simulink model "PROGRAM_COUNTER_05_SS"  (R2022a)
settings: Solver=VariableStepAuto  StartTime=0.0  StopTime=10.0  RelTol=1e-3
undefined symbols (not defined in the file or in its folder): xc7z010iclg225
libraries: hdlBasic x1928, hlsBasic x1, vmcUtilities x1
(part 3 of 12)

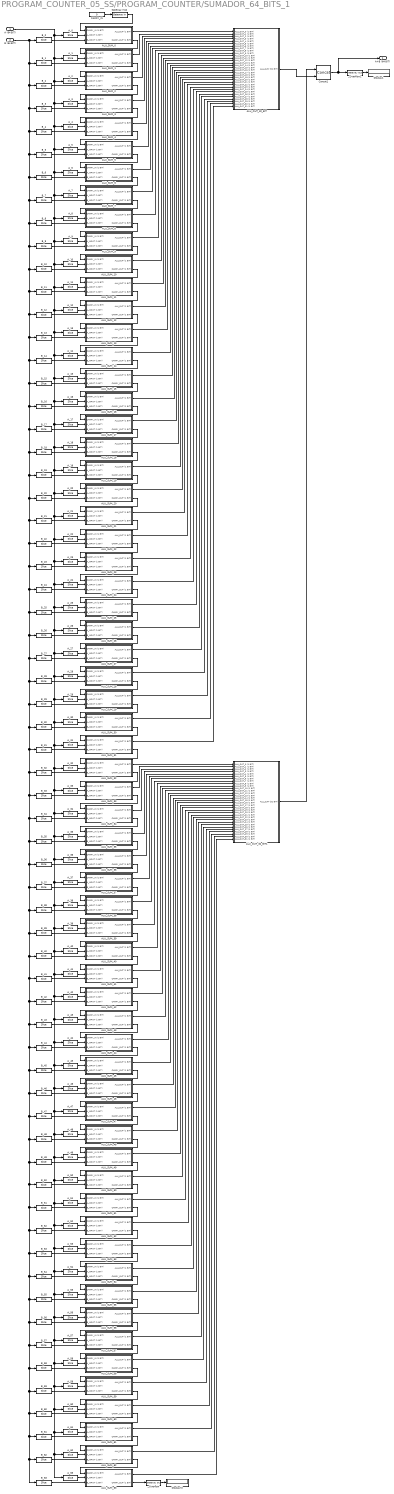
== system PROGRAM_COUNTER_05_SS/PROGRAM_COUNTER/SUMADOR_64_BITS_1 ==
  A (64 BIT) : Inport
  B (64 BIT) : Inport  Port=2
  ALU_OUT_32_BIT : Subsystem
  ALU_OUT_32_BIT1 : Subsystem
  ALU_SUM_0 : Subsystem
  ALU_SUM_1 : Subsystem
  ALU_SUM_10 : Subsystem
  ALU_SUM_11 : Subsystem
  ALU_SUM_12 : Subsystem
  ALU_SUM_13 : Subsystem
  ALU_SUM_14 : Subsystem
  ALU_SUM_15 : Subsystem
  ALU_SUM_16 : Subsystem
  ALU_SUM_17 : Subsystem
  ALU_SUM_18 : Subsystem
  ALU_SUM_19 : Subsystem
  ALU_SUM_2 : Subsystem
  ALU_SUM_20 : Subsystem
  ALU_SUM_21 : Subsystem
  ALU_SUM_22 : Subsystem
  ALU_SUM_23 : Subsystem
  ALU_SUM_24 : Subsystem
  ALU_SUM_25 : Subsystem
  ALU_SUM_26 : Subsystem
  ALU_SUM_27 : Subsystem
  ALU_SUM_28 : Subsystem
  ALU_SUM_29 : Subsystem
  ALU_SUM_3 : Subsystem
  ALU_SUM_30 : Subsystem
  ALU_SUM_31 : Subsystem
  ALU_SUM_32 : Subsystem
  ALU_SUM_33 : Subsystem
  ALU_SUM_34 : Subsystem
  ALU_SUM_35 : Subsystem
  ALU_SUM_36 : Subsystem
  ALU_SUM_37 : Subsystem
  ALU_SUM_38 : Subsystem
  ALU_SUM_39 : Subsystem
  ALU_SUM_4 : Subsystem
  ALU_SUM_40 : Subsystem
  ALU_SUM_41 : Subsystem
  ALU_SUM_42 : Subsystem
  ALU_SUM_43 : Subsystem
  ALU_SUM_44 : Subsystem
  ALU_SUM_45 : Subsystem
  ALU_SUM_46 : Subsystem
  ALU_SUM_47 : Subsystem
  ALU_SUM_48 : Subsystem
  ALU_SUM_49 : Subsystem
  ALU_SUM_5 : Subsystem
  ALU_SUM_50 : Subsystem
  ALU_SUM_51 : Subsystem
  ALU_SUM_52 : Subsystem
  ALU_SUM_53 : Subsystem
  ALU_SUM_54 : Subsystem
  ALU_SUM_55 : Subsystem
  ALU_SUM_56 : Subsystem
  ALU_SUM_57 : Subsystem
  ALU_SUM_58 : Subsystem
  ALU_SUM_59 : Subsystem
  ALU_SUM_6 : Subsystem
  ALU_SUM_60 : Subsystem
  ALU_SUM_61 : Subsystem
  ALU_SUM_62 : Subsystem
  ALU_SUM_63 : Subsystem
  ALU_SUM_7 : Subsystem
  ALU_SUM_8 : Subsystem
  ALU_SUM_9 : Subsystem
  A_0 : hdlBasic/Slice  nbits=1  boolean_output=off  mode=Lower Bit Location + Width  bit1=-3  base1=MSB of Input  bit0=0  base0=LSB of Input  XmcBlockStatus=1  maskContainerNames=group1  block_type=slice  block_config=sysgen:Slice_config
  A_1 : hdlBasic/Slice  nbits=1  boolean_output=off  mode=Lower Bit Location + Width  bit1=-2  base1=MSB of Input  bit0=1  base0=LSB of Input  XmcBlockStatus=1  maskContainerNames=group1  block_type=slice  block_config=sysgen:Slice_config
  A_10 : hdlBasic/Slice  nbits=1  boolean_output=off  mode=Lower Bit Location + Width  bit1=-1  base1=MSB of Input  bit0=10  base0=LSB of Input  XmcBlockStatus=1  maskContainerNames=group1  block_type=slice  block_config=sysgen:Slice_config
  A_11 : hdlBasic/Slice  nbits=1  boolean_output=off  mode=Lower Bit Location + Width  bit1=-3  base1=MSB of Input  bit0=11  base0=LSB of Input  XmcBlockStatus=1  maskContainerNames=group1  block_type=slice  block_config=sysgen:Slice_config
  A_12 : hdlBasic/Slice  nbits=1  boolean_output=off  mode=Lower Bit Location + Width  bit1=-2  base1=MSB of Input  bit0=12  base0=LSB of Input  XmcBlockStatus=1  maskContainerNames=group1  block_type=slice  block_config=sysgen:Slice_config
  A_13 : hdlBasic/Slice  nbits=1  boolean_output=off  mode=Lower Bit Location + Width  bit1=-1  base1=MSB of Input  bit0=13  base0=LSB of Input  XmcBlockStatus=1  maskContainerNames=group1  block_type=slice  block_config=sysgen:Slice_config
  A_14 : hdlBasic/Slice  nbits=1  boolean_output=off  mode=Lower Bit Location + Width  bit1=-1  base1=MSB of Input  bit0=14  base0=LSB of Input  XmcBlockStatus=1  maskContainerNames=group1  block_type=slice  block_config=sysgen:Slice_config
  A_15 : hdlBasic/Slice  nbits=1  boolean_output=off  mode=Lower Bit Location + Width  bit1=-3  base1=MSB of Input  bit0=15  base0=LSB of Input  XmcBlockStatus=1  maskContainerNames=group1  block_type=slice  block_config=sysgen:Slice_config
  A_16 : hdlBasic/Slice  nbits=1  boolean_output=off  mode=Lower Bit Location + Width  bit1=-2  base1=MSB of Input  bit0=16  base0=LSB of Input  XmcBlockStatus=1  maskContainerNames=group1  block_type=slice  block_config=sysgen:Slice_config
  A_17 : hdlBasic/Slice  nbits=1  boolean_output=off  mode=Lower Bit Location + Width  bit1=-1  base1=MSB of Input  bit0=17  base0=LSB of Input  XmcBlockStatus=1  maskContainerNames=group1  block_type=slice  block_config=sysgen:Slice_config
  A_18 : hdlBasic/Slice  nbits=1  boolean_output=off  mode=Lower Bit Location + Width  bit1=-1  base1=MSB of Input  bit0=18  base0=LSB of Input  XmcBlockStatus=1  maskContainerNames=group1  block_type=slice  block_config=sysgen:Slice_config
  A_19 : hdlBasic/Slice  nbits=1  boolean_output=off  mode=Lower Bit Location + Width  bit1=-3  base1=MSB of Input  bit0=19  base0=LSB of Input  XmcBlockStatus=1  maskContainerNames=group1  block_type=slice  block_config=sysgen:Slice_config
  A_2 : hdlBasic/Slice  nbits=1  boolean_output=off  mode=Lower Bit Location + Width  bit1=-1  base1=MSB of Input  bit0=2  base0=LSB of Input  XmcBlockStatus=1  maskContainerNames=group1  block_type=slice  block_config=sysgen:Slice_config
  A_20 : hdlBasic/Slice  nbits=1  boolean_output=off  mode=Lower Bit Location + Width  bit1=-2  base1=MSB of Input  bit0=20  base0=LSB of Input  XmcBlockStatus=1  maskContainerNames=group1  block_type=slice  block_config=sysgen:Slice_config
  A_21 : hdlBasic/Slice  nbits=1  boolean_output=off  mode=Lower Bit Location + Width  bit1=-1  base1=MSB of Input  bit0=21  base0=LSB of Input  XmcBlockStatus=1  maskContainerNames=group1  block_type=slice  block_config=sysgen:Slice_config
  A_22 : hdlBasic/Slice  nbits=1  boolean_output=off  mode=Lower Bit Location + Width  bit1=-1  base1=MSB of Input  bit0=22  base0=LSB of Input  XmcBlockStatus=1  maskContainerNames=group1  block_type=slice  block_config=sysgen:Slice_config
  A_23 : hdlBasic/Slice  nbits=1  boolean_output=off  mode=Lower Bit Location + Width  bit1=-3  base1=MSB of Input  bit0=23  base0=LSB of Input  XmcBlockStatus=1  maskContainerNames=group1  block_type=slice  block_config=sysgen:Slice_config
  A_24 : hdlBasic/Slice  nbits=1  boolean_output=off  mode=Lower Bit Location + Width  bit1=-2  base1=MSB of Input  bit0=24  base0=LSB of Input  XmcBlockStatus=1  maskContainerNames=group1  block_type=slice  block_config=sysgen:Slice_config
  A_25 : hdlBasic/Slice  nbits=1  boolean_output=off  mode=Lower Bit Location + Width  bit1=-1  base1=MSB of Input  bit0=25  base0=LSB of Input  XmcBlockStatus=1  maskContainerNames=group1  block_type=slice  block_config=sysgen:Slice_config
  A_26 : hdlBasic/Slice  nbits=1  boolean_output=off  mode=Lower Bit Location + Width  bit1=-1  base1=MSB of Input  bit0=26  base0=LSB of Input  XmcBlockStatus=1  maskContainerNames=group1  block_type=slice  block_config=sysgen:Slice_config
  A_27 : hdlBasic/Slice  nbits=1  boolean_output=off  mode=Lower Bit Location + Width  bit1=-3  base1=MSB of Input  bit0=27  base0=LSB of Input  XmcBlockStatus=1  maskContainerNames=group1  block_type=slice  block_config=sysgen:Slice_config
  A_28 : hdlBasic/Slice  nbits=1  boolean_output=off  mode=Lower Bit Location + Width  bit1=-2  base1=MSB of Input  bit0=28  base0=LSB of Input  XmcBlockStatus=1  maskContainerNames=group1  block_type=slice  block_config=sysgen:Slice_config
  A_29 : hdlBasic/Slice  nbits=1  boolean_output=off  mode=Lower Bit Location + Width  bit1=-1  base1=MSB of Input  bit0=29  base0=LSB of Input  XmcBlockStatus=1  maskContainerNames=group1  block_type=slice  block_config=sysgen:Slice_config
  A_3 : hdlBasic/Slice  nbits=1  boolean_output=off  mode=Lower Bit Location + Width  bit1=-3  base1=MSB of Input  bit0=3  base0=LSB of Input  XmcBlockStatus=1  maskContainerNames=group1  block_type=slice  block_config=sysgen:Slice_config
  A_30 : hdlBasic/Slice  nbits=1  boolean_output=off  mode=Lower Bit Location + Width  bit1=-1  base1=MSB of Input  bit0=30  base0=LSB of Input  XmcBlockStatus=1  maskContainerNames=group1  block_type=slice  block_config=sysgen:Slice_config
  A_31 : hdlBasic/Slice  nbits=1  boolean_output=off  mode=Lower Bit Location + Width  bit1=-3  base1=MSB of Input  bit0=31  base0=LSB of Input  XmcBlockStatus=1  maskContainerNames=group1  block_type=slice  block_config=sysgen:Slice_config
  A_32 : hdlBasic/Slice  nbits=1  boolean_output=off  mode=Lower Bit Location + Width  bit1=-1  base1=MSB of Input  bit0=32  base0=LSB of Input  XmcBlockStatus=1  maskContainerNames=group1  block_type=slice  block_config=sysgen:Slice_config
  A_33 : hdlBasic/Slice  nbits=1  boolean_output=off  mode=Lower Bit Location + Width  bit1=-3  base1=MSB of Input  bit0=33  base0=LSB of Input  XmcBlockStatus=1  maskContainerNames=group1  block_type=slice  block_config=sysgen:Slice_config
  A_34 : hdlBasic/Slice  nbits=1  boolean_output=off  mode=Lower Bit Location + Width  bit1=-1  base1=MSB of Input  bit0=34  base0=LSB of Input  XmcBlockStatus=1  maskContainerNames=group1  block_type=slice  block_config=sysgen:Slice_config
  A_35 : hdlBasic/Slice  nbits=1  boolean_output=off  mode=Lower Bit Location + Width  bit1=-3  base1=MSB of Input  bit0=35  base0=LSB of Input  XmcBlockStatus=1  maskContainerNames=group1  block_type=slice  block_config=sysgen:Slice_config
  A_36 : hdlBasic/Slice  nbits=1  boolean_output=off  mode=Lower Bit Location + Width  bit1=-1  base1=MSB of Input  bit0=36  base0=LSB of Input  XmcBlockStatus=1  maskContainerNames=group1  block_type=slice  block_config=sysgen:Slice_config
  A_37 : hdlBasic/Slice  nbits=1  boolean_output=off  mode=Lower Bit Location + Width  bit1=-3  base1=MSB of Input  bit0=37  base0=LSB of Input  XmcBlockStatus=1  maskContainerNames=group1  block_type=slice  block_config=sysgen:Slice_config
  A_38 : hdlBasic/Slice  nbits=1  boolean_output=off  mode=Lower Bit Location + Width  bit1=-1  base1=MSB of Input  bit0=38  base0=LSB of Input  XmcBlockStatus=1  maskContainerNames=group1  block_type=slice  block_config=sysgen:Slice_config
  A_39 : hdlBasic/Slice  nbits=1  boolean_output=off  mode=Lower Bit Location + Width  bit1=-3  base1=MSB of Input  bit0=39  base0=LSB of Input  XmcBlockStatus=1  maskContainerNames=group1  block_type=slice  block_config=sysgen:Slice_config
  A_4 : hdlBasic/Slice  nbits=1  boolean_output=off  mode=Lower Bit Location + Width  bit1=-2  base1=MSB of Input  bit0=4  base0=LSB of Input  XmcBlockStatus=1  maskContainerNames=group1  block_type=slice  block_config=sysgen:Slice_config
  A_40 : hdlBasic/Slice  nbits=1  boolean_output=off  mode=Lower Bit Location + Width  bit1=-1  base1=MSB of Input  bit0=40  base0=LSB of Input  XmcBlockStatus=1  maskContainerNames=group1  block_type=slice  block_config=sysgen:Slice_config
  A_41 : hdlBasic/Slice  nbits=1  boolean_output=off  mode=Lower Bit Location + Width  bit1=-3  base1=MSB of Input  bit0=41  base0=LSB of Input  XmcBlockStatus=1  maskContainerNames=group1  block_type=slice  block_config=sysgen:Slice_config
  A_42 : hdlBasic/Slice  nbits=1  boolean_output=off  mode=Lower Bit Location + Width  bit1=-1  base1=MSB of Input  bit0=42  base0=LSB of Input  XmcBlockStatus=1  maskContainerNames=group1  block_type=slice  block_config=sysgen:Slice_config
  A_43 : hdlBasic/Slice  nbits=1  boolean_output=off  mode=Lower Bit Location + Width  bit1=-3  base1=MSB of Input  bit0=43  base0=LSB of Input  XmcBlockStatus=1  maskContainerNames=group1  block_type=slice  block_config=sysgen:Slice_config
  A_44 : hdlBasic/Slice  nbits=1  boolean_output=off  mode=Lower Bit Location + Width  bit1=-1  base1=MSB of Input  bit0=44  base0=LSB of Input  XmcBlockStatus=1  maskContainerNames=group1  block_type=slice  block_config=sysgen:Slice_config
  A_45 : hdlBasic/Slice  nbits=1  boolean_output=off  mode=Lower Bit Location + Width  bit1=-3  base1=MSB of Input  bit0=45  base0=LSB of Input  XmcBlockStatus=1  maskContainerNames=group1  block_type=slice  block_config=sysgen:Slice_config
  A_46 : hdlBasic/Slice  nbits=1  boolean_output=off  mode=Lower Bit Location + Width  bit1=-1  base1=MSB of Input  bit0=46  base0=LSB of Input  XmcBlockStatus=1  maskContainerNames=group1  block_type=slice  block_config=sysgen:Slice_config
  A_47 : hdlBasic/Slice  nbits=1  boolean_output=off  mode=Lower Bit Location + Width  bit1=-3  base1=MSB of Input  bit0=47  base0=LSB of Input  XmcBlockStatus=1  maskContainerNames=group1  block_type=slice  block_config=sysgen:Slice_config
  A_48 : hdlBasic/Slice  nbits=1  boolean_output=off  mode=Lower Bit Location + Width  bit1=-1  base1=MSB of Input  bit0=48  base0=LSB of Input  XmcBlockStatus=1  maskContainerNames=group1  block_type=slice  block_config=sysgen:Slice_config
  A_49 : hdlBasic/Slice  nbits=1  boolean_output=off  mode=Lower Bit Location + Width  bit1=-3  base1=MSB of Input  bit0=49  base0=LSB of Input  XmcBlockStatus=1  maskContainerNames=group1  block_type=slice  block_config=sysgen:Slice_config
  A_5 : hdlBasic/Slice  nbits=1  boolean_output=off  mode=Lower Bit Location + Width  bit1=-1  base1=MSB of Input  bit0=5  base0=LSB of Input  XmcBlockStatus=1  maskContainerNames=group1  block_type=slice  block_config=sysgen:Slice_config
  A_50 : hdlBasic/Slice  nbits=1  boolean_output=off  mode=Lower Bit Location + Width  bit1=-1  base1=MSB of Input  bit0=50  base0=LSB of Input  XmcBlockStatus=1  maskContainerNames=group1  block_type=slice  block_config=sysgen:Slice_config
  A_51 : hdlBasic/Slice  nbits=1  boolean_output=off  mode=Lower Bit Location + Width  bit1=-3  base1=MSB of Input  bit0=51  base0=LSB of Input  XmcBlockStatus=1  maskContainerNames=group1  block_type=slice  block_config=sysgen:Slice_config
  A_52 : hdlBasic/Slice  nbits=1  boolean_output=off  mode=Lower Bit Location + Width  bit1=-1  base1=MSB of Input  bit0=52  base0=LSB of Input  XmcBlockStatus=1  maskContainerNames=group1  block_type=slice  block_config=sysgen:Slice_config
  A_53 : hdlBasic/Slice  nbits=1  boolean_output=off  mode=Lower Bit Location + Width  bit1=-3  base1=MSB of Input  bit0=53  base0=LSB of Input  XmcBlockStatus=1  maskContainerNames=group1  block_type=slice  block_config=sysgen:Slice_config
  A_54 : hdlBasic/Slice  nbits=1  boolean_output=off  mode=Lower Bit Location + Width  bit1=-1  base1=MSB of Input  bit0=54  base0=LSB of Input  XmcBlockStatus=1  maskContainerNames=group1  block_type=slice  block_config=sysgen:Slice_config
  A_55 : hdlBasic/Slice  nbits=1  boolean_output=off  mode=Lower Bit Location + Width  bit1=-3  base1=MSB of Input  bit0=55  base0=LSB of Input  XmcBlockStatus=1  maskContainerNames=group1  block_type=slice  block_config=sysgen:Slice_config
  A_56 : hdlBasic/Slice  nbits=1  boolean_output=off  mode=Lower Bit Location + Width  bit1=-1  base1=MSB of Input  bit0=56  base0=LSB of Input  XmcBlockStatus=1  maskContainerNames=group1  block_type=slice  block_config=sysgen:Slice_config
  A_57 : hdlBasic/Slice  nbits=1  boolean_output=off  mode=Lower Bit Location + Width  bit1=-3  base1=MSB of Input  bit0=57  base0=LSB of Input  XmcBlockStatus=1  maskContainerNames=group1  block_type=slice  block_config=sysgen:Slice_config
  A_58 : hdlBasic/Slice  nbits=1  boolean_output=off  mode=Lower Bit Location + Width  bit1=-1  base1=MSB of Input  bit0=58  base0=LSB of Input  XmcBlockStatus=1  maskContainerNames=group1  block_type=slice  block_config=sysgen:Slice_config
  A_59 : hdlBasic/Slice  nbits=1  boolean_output=off  mode=Lower Bit Location + Width  bit1=-3  base1=MSB of Input  bit0=59  base0=LSB of Input  XmcBlockStatus=1  maskContainerNames=group1  block_type=slice  block_config=sysgen:Slice_config
  A_6 : hdlBasic/Slice  nbits=1  boolean_output=off  mode=Lower Bit Location + Width  bit1=-1  base1=MSB of Input  bit0=6  base0=LSB of Input  XmcBlockStatus=1  maskContainerNames=group1  block_type=slice  block_config=sysgen:Slice_config
  A_60 : hdlBasic/Slice  nbits=1  boolean_output=off  mode=Lower Bit Location + Width  bit1=-1  base1=MSB of Input  bit0=60  base0=LSB of Input  XmcBlockStatus=1  maskContainerNames=group1  block_type=slice  block_config=sysgen:Slice_config
  A_61 : hdlBasic/Slice  nbits=1  boolean_output=off  mode=Lower Bit Location + Width  bit1=-3  base1=MSB of Input  bit0=61  base0=LSB of Input  XmcBlockStatus=1  maskContainerNames=group1  block_type=slice  block_config=sysgen:Slice_config
  A_62 : hdlBasic/Slice  nbits=1  boolean_output=off  mode=Lower Bit Location + Width  bit1=-1  base1=MSB of Input  bit0=62  base0=LSB of Input  XmcBlockStatus=1  maskContainerNames=group1  block_type=slice  block_config=sysgen:Slice_config
  A_63 : hdlBasic/Slice  nbits=1  boolean_output=off  mode=Lower Bit Location + Width  bit1=-3  base1=MSB of Input  bit0=63  base0=LSB of Input  XmcBlockStatus=1  maskContainerNames=group1  block_type=slice  block_config=sysgen:Slice_config
  A_7 : hdlBasic/Slice  nbits=1  boolean_output=off  mode=Lower Bit Location + Width  bit1=-3  base1=MSB of Input  bit0=7  base0=LSB of Input  XmcBlockStatus=1  maskContainerNames=group1  block_type=slice  block_config=sysgen:Slice_config
  A_8 : hdlBasic/Slice  nbits=1  boolean_output=off  mode=Lower Bit Location + Width  bit1=-2  base1=MSB of Input  bit0=8  base0=LSB of Input  XmcBlockStatus=1  maskContainerNames=group1  block_type=slice  block_config=sysgen:Slice_config
  A_9 : hdlBasic/Slice  nbits=1  boolean_output=off  mode=Lower Bit Location + Width  bit1=-1  base1=MSB of Input  bit0=9  base0=LSB of Input  XmcBlockStatus=1  maskContainerNames=group1  block_type=slice  block_config=sysgen:Slice_config
  B_0 : hdlBasic/Slice  nbits=1  boolean_output=off  mode=Lower Bit Location + Width  bit1=-3  base1=MSB of Input  bit0=0  base0=LSB of Input  XmcBlockStatus=1  maskContainerNames=group1  block_type=slice  block_config=sysgen:Slice_config
  B_1 : hdlBasic/Slice  nbits=1  boolean_output=off  mode=Lower Bit Location + Width  bit1=-3  base1=MSB of Input  bit0=1  base0=LSB of Input  XmcBlockStatus=1  maskContainerNames=group1  block_type=slice  block_config=sysgen:Slice_config
  B_10 : hdlBasic/Slice  nbits=1  boolean_output=off  mode=Lower Bit Location + Width  bit1=-3  base1=MSB of Input  bit0=10  base0=LSB of Input  XmcBlockStatus=1  maskContainerNames=group1  block_type=slice  block_config=sysgen:Slice_config
  B_11 : hdlBasic/Slice  nbits=1  boolean_output=off  mode=Lower Bit Location + Width  bit1=-3  base1=MSB of Input  bit0=11  base0=LSB of Input  XmcBlockStatus=1  maskContainerNames=group1  block_type=slice  block_config=sysgen:Slice_config
  B_12 : hdlBasic/Slice  nbits=1  boolean_output=off  mode=Lower Bit Location + Width  bit1=-3  base1=MSB of Input  bit0=12  base0=LSB of Input  XmcBlockStatus=1  maskContainerNames=group1  block_type=slice  block_config=sysgen:Slice_config
  B_13 : hdlBasic/Slice  nbits=1  boolean_output=off  mode=Lower Bit Location + Width  bit1=-3  base1=MSB of Input  bit0=13  base0=LSB of Input  XmcBlockStatus=1  maskContainerNames=group1  block_type=slice  block_config=sysgen:Slice_config
  B_14 : hdlBasic/Slice  nbits=1  boolean_output=off  mode=Lower Bit Location + Width  bit1=-3  base1=MSB of Input  bit0=14  base0=LSB of Input  XmcBlockStatus=1  maskContainerNames=group1  block_type=slice  block_config=sysgen:Slice_config
  B_15 : hdlBasic/Slice  nbits=1  boolean_output=off  mode=Lower Bit Location + Width  bit1=-3  base1=MSB of Input  bit0=15  base0=LSB of Input  XmcBlockStatus=1  maskContainerNames=group1  block_type=slice  block_config=sysgen:Slice_config
  B_16 : hdlBasic/Slice  nbits=1  boolean_output=off  mode=Lower Bit Location + Width  bit1=-3  base1=MSB of Input  bit0=16  base0=LSB of Input  XmcBlockStatus=1  maskContainerNames=group1  block_type=slice  block_config=sysgen:Slice_config
  B_17 : hdlBasic/Slice  nbits=1  boolean_output=off  mode=Lower Bit Location + Width  bit1=-3  base1=MSB of Input  bit0=17  base0=LSB of Input  XmcBlockStatus=1  maskContainerNames=group1  block_type=slice  block_config=sysgen:Slice_config
  B_18 : hdlBasic/Slice  nbits=1  boolean_output=off  mode=Lower Bit Location + Width  bit1=-3  base1=MSB of Input  bit0=18  base0=LSB of Input  XmcBlockStatus=1  maskContainerNames=group1  block_type=slice  block_config=sysgen:Slice_config
  B_19 : hdlBasic/Slice  nbits=1  boolean_output=off  mode=Lower Bit Location + Width  bit1=-3  base1=MSB of Input  bit0=19  base0=LSB of Input  XmcBlockStatus=1  maskContainerNames=group1  block_type=slice  block_config=sysgen:Slice_config
  B_2 : hdlBasic/Slice  nbits=1  boolean_output=off  mode=Lower Bit Location + Width  bit1=-3  base1=MSB of Input  bit0=2  base0=LSB of Input  XmcBlockStatus=1  maskContainerNames=group1  block_type=slice  block_config=sysgen:Slice_config
  B_20 : hdlBasic/Slice  nbits=1  boolean_output=off  mode=Lower Bit Location + Width  bit1=-3  base1=MSB of Input  bit0=20  base0=LSB of Input  XmcBlockStatus=1  maskContainerNames=group1  block_type=slice  block_config=sysgen:Slice_config
  B_21 : hdlBasic/Slice  nbits=1  boolean_output=off  mode=Lower Bit Location + Width  bit1=-3  base1=MSB of Input  bit0=21  base0=LSB of Input  XmcBlockStatus=1  maskContainerNames=group1  block_type=slice  block_config=sysgen:Slice_config
  B_22 : hdlBasic/Slice  nbits=1  boolean_output=off  mode=Lower Bit Location + Width  bit1=-3  base1=MSB of Input  bit0=22  base0=LSB of Input  XmcBlockStatus=1  maskContainerNames=group1  block_type=slice  block_config=sysgen:Slice_config
  B_23 : hdlBasic/Slice  nbits=1  boolean_output=off  mode=Lower Bit Location + Width  bit1=-3  base1=MSB of Input  bit0=23  base0=LSB of Input  XmcBlockStatus=1  maskContainerNames=group1  block_type=slice  block_config=sysgen:Slice_config
  B_24 : hdlBasic/Slice  nbits=1  boolean_output=off  mode=Lower Bit Location + Width  bit1=-3  base1=MSB of Input  bit0=24  base0=LSB of Input  XmcBlockStatus=1  maskContainerNames=group1  block_type=slice  block_config=sysgen:Slice_config
  B_25 : hdlBasic/Slice  nbits=1  boolean_output=off  mode=Lower Bit Location + Width  bit1=-3  base1=MSB of Input  bit0=25  base0=LSB of Input  XmcBlockStatus=1  maskContainerNames=group1  block_type=slice  block_config=sysgen:Slice_config
  B_26 : hdlBasic/Slice  nbits=1  boolean_output=off  mode=Lower Bit Location + Width  bit1=-3  base1=MSB of Input  bit0=26  base0=LSB of Input  XmcBlockStatus=1  maskContainerNames=group1  block_type=slice  block_config=sysgen:Slice_config
  B_27 : hdlBasic/Slice  nbits=1  boolean_output=off  mode=Lower Bit Location + Width  bit1=-3  base1=MSB of Input  bit0=27  base0=LSB of Input  XmcBlockStatus=1  maskContainerNames=group1  block_type=slice  block_config=sysgen:Slice_config
  B_28 : hdlBasic/Slice  nbits=1  boolean_output=off  mode=Lower Bit Location + Width  bit1=-3  base1=MSB of Input  bit0=28  base0=LSB of Input  XmcBlockStatus=1  maskContainerNames=group1  block_type=slice  block_config=sysgen:Slice_config
  B_29 : hdlBasic/Slice  nbits=1  boolean_output=off  mode=Lower Bit Location + Width  bit1=-3  base1=MSB of Input  bit0=29  base0=LSB of Input  XmcBlockStatus=1  maskContainerNames=group1  block_type=slice  block_config=sysgen:Slice_config
  B_3 : hdlBasic/Slice  nbits=1  boolean_output=off  mode=Lower Bit Location + Width  bit1=-3  base1=MSB of Input  bit0=3  base0=LSB of Input  XmcBlockStatus=1  maskContainerNames=group1  block_type=slice  block_config=sysgen:Slice_config
  B_30 : hdlBasic/Slice  nbits=1  boolean_output=off  mode=Lower Bit Location + Width  bit1=-3  base1=MSB of Input  bit0=30  base0=LSB of Input  XmcBlockStatus=1  maskContainerNames=group1  block_type=slice  block_config=sysgen:Slice_config
  B_31 : hdlBasic/Slice  nbits=1  boolean_output=off  mode=Lower Bit Location + Width  bit1=-3  base1=MSB of Input  bit0=31  base0=LSB of Input  XmcBlockStatus=1  maskContainerNames=group1  block_type=slice  block_config=sysgen:Slice_config
  B_32 : hdlBasic/Slice  nbits=1  boolean_output=off  mode=Lower Bit Location + Width  bit1=-3  base1=MSB of Input  bit0=32  base0=LSB of Input  XmcBlockStatus=1  maskContainerNames=group1  block_type=slice  block_config=sysgen:Slice_config
  B_33 : hdlBasic/Slice  nbits=1  boolean_output=off  mode=Lower Bit Location + Width  bit1=-3  base1=MSB of Input  bit0=33  base0=LSB of Input  XmcBlockStatus=1  maskContainerNames=group1  block_type=slice  block_config=sysgen:Slice_config
  B_34 : hdlBasic/Slice  nbits=1  boolean_output=off  mode=Lower Bit Location + Width  bit1=-3  base1=MSB of Input  bit0=34  base0=LSB of Input  XmcBlockStatus=1  maskContainerNames=group1  block_type=slice  block_config=sysgen:Slice_config
  B_35 : hdlBasic/Slice  nbits=1  boolean_output=off  mode=Lower Bit Location + Width  bit1=-3  base1=MSB of Input  bit0=35  base0=LSB of Input  XmcBlockStatus=1  maskContainerNames=group1  block_type=slice  block_config=sysgen:Slice_config
  B_36 : hdlBasic/Slice  nbits=1  boolean_output=off  mode=Lower Bit Location + Width  bit1=-3  base1=MSB of Input  bit0=36  base0=LSB of Input  XmcBlockStatus=1  maskContainerNames=group1  block_type=slice  block_config=sysgen:Slice_config
  B_37 : hdlBasic/Slice  nbits=1  boolean_output=off  mode=Lower Bit Location + Width  bit1=-3  base1=MSB of Input  bit0=37  base0=LSB of Input  XmcBlockStatus=1  maskContainerNames=group1  block_type=slice  block_config=sysgen:Slice_config
  B_38 : hdlBasic/Slice  nbits=1  boolean_output=off  mode=Lower Bit Location + Width  bit1=-3  base1=MSB of Input  bit0=38  base0=LSB of Input  XmcBlockStatus=1  maskContainerNames=group1  block_type=slice  block_config=sysgen:Slice_config
  B_39 : hdlBasic/Slice  nbits=1  boolean_output=off  mode=Lower Bit Location + Width  bit1=-3  base1=MSB of Input  bit0=39  base0=LSB of Input  XmcBlockStatus=1  maskContainerNames=group1  block_type=slice  block_config=sysgen:Slice_config
  B_4 : hdlBasic/Slice  nbits=1  boolean_output=off  mode=Lower Bit Location + Width  bit1=-3  base1=MSB of Input  bit0=4  base0=LSB of Input  XmcBlockStatus=1  maskContainerNames=group1  block_type=slice  block_config=sysgen:Slice_config
  B_40 : hdlBasic/Slice  nbits=1  boolean_output=off  mode=Lower Bit Location + Width  bit1=-3  base1=MSB of Input  bit0=40  base0=LSB of Input  XmcBlockStatus=1  maskContainerNames=group1  block_type=slice  block_config=sysgen:Slice_config
  B_41 : hdlBasic/Slice  nbits=1  boolean_output=off  mode=Lower Bit Location + Width  bit1=-3  base1=MSB of Input  bit0=41  base0=LSB of Input  XmcBlockStatus=1  maskContainerNames=group1  block_type=slice  block_config=sysgen:Slice_config
  B_42 : hdlBasic/Slice  nbits=1  boolean_output=off  mode=Lower Bit Location + Width  bit1=-3  base1=MSB of Input  bit0=42  base0=LSB of Input  XmcBlockStatus=1  maskContainerNames=group1  block_type=slice  block_config=sysgen:Slice_config
  B_43 : hdlBasic/Slice  nbits=1  boolean_output=off  mode=Lower Bit Location + Width  bit1=-3  base1=MSB of Input  bit0=43  base0=LSB of Input  XmcBlockStatus=1  maskContainerNames=group1  block_type=slice  block_config=sysgen:Slice_config
  B_44 : hdlBasic/Slice  nbits=1  boolean_output=off  mode=Lower Bit Location + Width  bit1=-3  base1=MSB of Input  bit0=44  base0=LSB of Input  XmcBlockStatus=1  maskContainerNames=group1  block_type=slice  block_config=sysgen:Slice_config
  B_45 : hdlBasic/Slice  nbits=1  boolean_output=off  mode=Lower Bit Location + Width  bit1=-3  base1=MSB of Input  bit0=45  base0=LSB of Input  XmcBlockStatus=1  maskContainerNames=group1  block_type=slice  block_config=sysgen:Slice_config
  B_46 : hdlBasic/Slice  nbits=1  boolean_output=off  mode=Lower Bit Location + Width  bit1=-3  base1=MSB of Input  bit0=46  base0=LSB of Input  XmcBlockStatus=1  maskContainerNames=group1  block_type=slice  block_config=sysgen:Slice_config
  B_47 : hdlBasic/Slice  nbits=1  boolean_output=off  mode=Lower Bit Location + Width  bit1=-3  base1=MSB of Input  bit0=47  base0=LSB of Input  XmcBlockStatus=1  maskContainerNames=group1  block_type=slice  block_config=sysgen:Slice_config
  B_48 : hdlBasic/Slice  nbits=1  boolean_output=off  mode=Lower Bit Location + Width  bit1=-3  base1=MSB of Input  bit0=48  base0=LSB of Input  XmcBlockStatus=1  maskContainerNames=group1  block_type=slice  block_config=sysgen:Slice_config
  B_49 : hdlBasic/Slice  nbits=1  boolean_output=off  mode=Lower Bit Location + Width  bit1=-3  base1=MSB of Input  bit0=49  base0=LSB of Input  XmcBlockStatus=1  maskContainerNames=group1  block_type=slice  block_config=sysgen:Slice_config
  B_5 : hdlBasic/Slice  nbits=1  boolean_output=off  mode=Lower Bit Location + Width  bit1=-3  base1=MSB of Input  bit0=5  base0=LSB of Input  XmcBlockStatus=1  maskContainerNames=group1  block_type=slice  block_config=sysgen:Slice_config
  B_50 : hdlBasic/Slice  nbits=1  boolean_output=off  mode=Lower Bit Location + Width  bit1=-3  base1=MSB of Input  bit0=50  base0=LSB of Input  XmcBlockStatus=1  maskContainerNames=group1  block_type=slice  block_config=sysgen:Slice_config
  B_51 : hdlBasic/Slice  nbits=1  boolean_output=off  mode=Lower Bit Location + Width  bit1=-3  base1=MSB of Input  bit0=51  base0=LSB of Input  XmcBlockStatus=1  maskContainerNames=group1  block_type=slice  block_config=sysgen:Slice_config
  B_52 : hdlBasic/Slice  nbits=1  boolean_output=off  mode=Lower Bit Location + Width  bit1=-3  base1=MSB of Input  bit0=52  base0=LSB of Input  XmcBlockStatus=1  maskContainerNames=group1  block_type=slice  block_config=sysgen:Slice_config
  B_53 : hdlBasic/Slice  nbits=1  boolean_output=off  mode=Lower Bit Location + Width  bit1=-3  base1=MSB of Input  bit0=53  base0=LSB of Input  XmcBlockStatus=1  maskContainerNames=group1  block_type=slice  block_config=sysgen:Slice_config
  B_54 : hdlBasic/Slice  nbits=1  boolean_output=off  mode=Lower Bit Location + Width  bit1=-3  base1=MSB of Input  bit0=54  base0=LSB of Input  XmcBlockStatus=1  maskContainerNames=group1  block_type=slice  block_config=sysgen:Slice_config
  B_55 : hdlBasic/Slice  nbits=1  boolean_output=off  mode=Lower Bit Location + Width  bit1=-3  base1=MSB of Input  bit0=55  base0=LSB of Input  XmcBlockStatus=1  maskContainerNames=group1  block_type=slice  block_config=sysgen:Slice_config
  B_56 : hdlBasic/Slice  nbits=1  boolean_output=off  mode=Lower Bit Location + Width  bit1=-3  base1=MSB of Input  bit0=56  base0=LSB of Input  XmcBlockStatus=1  maskContainerNames=group1  block_type=slice  block_config=sysgen:Slice_config
  B_57 : hdlBasic/Slice  nbits=1  boolean_output=off  mode=Lower Bit Location + Width  bit1=-3  base1=MSB of Input  bit0=57  base0=LSB of Input  XmcBlockStatus=1  maskContainerNames=group1  block_type=slice  block_config=sysgen:Slice_config
  B_58 : hdlBasic/Slice  nbits=1  boolean_output=off  mode=Lower Bit Location + Width  bit1=-3  base1=MSB of Input  bit0=58  base0=LSB of Input  XmcBlockStatus=1  maskContainerNames=group1  block_type=slice  block_config=sysgen:Slice_config
  B_59 : hdlBasic/Slice  nbits=1  boolean_output=off  mode=Lower Bit Location + Width  bit1=-3  base1=MSB of Input  bit0=59  base0=LSB of Input  XmcBlockStatus=1  maskContainerNames=group1  block_type=slice  block_config=sysgen:Slice_config
  B_6 : hdlBasic/Slice  nbits=1  boolean_output=off  mode=Lower Bit Location + Width  bit1=-3  base1=MSB of Input  bit0=6  base0=LSB of Input  XmcBlockStatus=1  maskContainerNames=group1  block_type=slice  block_config=sysgen:Slice_config
  B_60 : hdlBasic/Slice  nbits=1  boolean_output=off  mode=Lower Bit Location + Width  bit1=-3  base1=MSB of Input  bit0=60  base0=LSB of Input  XmcBlockStatus=1  maskContainerNames=group1  block_type=slice  block_config=sysgen:Slice_config
  B_61 : hdlBasic/Slice  nbits=1  boolean_output=off  mode=Lower Bit Location + Width  bit1=-3  base1=MSB of Input  bit0=61  base0=LSB of Input  XmcBlockStatus=1  maskContainerNames=group1  block_type=slice  block_config=sysgen:Slice_config
  B_62 : hdlBasic/Slice  nbits=1  boolean_output=off  mode=Lower Bit Location + Width  bit1=-3  base1=MSB of Input  bit0=62  base0=LSB of Input  XmcBlockStatus=1  maskContainerNames=group1  block_type=slice  block_config=sysgen:Slice_config
  B_63 : hdlBasic/Slice  nbits=1  boolean_output=off  mode=Lower Bit Location + Width  bit1=-3  base1=MSB of Input  bit0=63  base0=LSB of Input  XmcBlockStatus=1  maskContainerNames=group1  block_type=slice  block_config=sysgen:Slice_config
  B_7 : hdlBasic/Slice  nbits=1  boolean_output=off  mode=Lower Bit Location + Width  bit1=-3  base1=MSB of Input  bit0=7  base0=LSB of Input  XmcBlockStatus=1  maskContainerNames=group1  block_type=slice  block_config=sysgen:Slice_config
  B_8 : hdlBasic/Slice  nbits=1  boolean_output=off  mode=Lower Bit Location + Width  bit1=-3  base1=MSB of Input  bit0=8  base0=LSB of Input  XmcBlockStatus=1  maskContainerNames=group1  block_type=slice  block_config=sysgen:Slice_config
  B_9 : hdlBasic/Slice  nbits=1  boolean_output=off  mode=Lower Bit Location + Width  bit1=-3  base1=MSB of Input  bit0=9  base0=LSB of Input  XmcBlockStatus=1  maskContainerNames=group1  block_type=slice  block_config=sysgen:Slice_config
  CARRY_IN : Constant  Value=0
  Concat1 : hdlBasic/Concat  num_inputs=2  XmcBlockStatus=1  maskContainerNames=group1  block_type=concat  block_config=sysgen:Concat_config
  Display1 : Display
  Display72 : Display
  Gateway In12 : hdlBasic/Gateway In  gui_display_data_type=Fixed-point  arith_type=Unsigned  n_bits=1  bin_pt=0  preci_type=Single  exp_width=8  frac_width=24  rows=1  columns=1  quantization="Round  (unbiased: +/- Inf)"  overflow=Saturate  period=1  UseAsADC=off  ADCChannel='1'  interface=None  automatic_assignment=on  address_offset=hex2dec('00')  intf_name=''  intf_description=''  default_value=0  timing_constraint=None  locs_specified=off  LOCs={}  io_standard={}  inherit_from_input=off  hdl_port=on  XmcBlockStatus=1  maskContainerNames=group4  block_type=gatewayin  block_config=sysgen:gateway_in_config  block_width_w=590  block_height_w=620  block_width=640  block_height=850
  _Overflow : hdlBasic/Gateway Out  inherit_from_input=off  hdl_port=on  rows=1  columns=1  UseAsDAC=off  DACChannel='1'  interface=None  automatic_assignment=on  address_offset=hex2dec('00')  intf_name=''  intf_description=''  timing_constraint=None  locs_specified=off  LOCs={}  io_standard={}  XmcBlockStatus=1  maskContainerNames=group4  block_type=gatewayout  block_config=sysgen:gateway_out_config  block_width_w=590  block_height_w=620  block_width=620  block_height=750
  _Overflow1 : hdlBasic/Gateway Out  inherit_from_input=off  hdl_port=on  rows=1  columns=1  UseAsDAC=off  DACChannel='1'  interface=None  automatic_assignment=on  address_offset=hex2dec('00')  intf_name=''  intf_description=''  timing_constraint=None  locs_specified=off  LOCs={}  io_standard={}  XmcBlockStatus=1  maskContainerNames=group4  block_type=gatewayout  block_config=sysgen:gateway_out_config  block_width_w=590  block_height_w=620  block_width=620  block_height=750
  A+B (64 BIT) : Outport
  wires:
  ALU_SUM_62/1(ALU_OUT (1 BIT)) -> ALU_OUT_32_BIT1/31(ALU_OUT_30 (1 BIT))
  ALU_SUM_61/2(CARRY_OUT (1 BIT)) -> ALU_SUM_62/1(CARRY_IN (1 BIT))
  A (64 BIT)/1 -> A_63/1, A_62/1, A_61/1, A_60/1, A_59/1, A_58/1, A_57/1, A_56/1, A_55/1, A_54/1, A_53/1, A_52/1, A_51/1, A_50/1, A_49/1, A_48/1, A_47/1, A_46/1, A_45/1, A_44/1, A_43/1, A_42/1, A_41/1, A_40/1, A_39/1, A_38/1, A_37/1, A_36/1, A_35/1, A_34/1, A_33/1, A_32/1, A_31/1, A_30/1, A_29/1, A_28/1, A_27/1, A_26/1, A_25/1, A_24/1, A_23/1, A_22/1, A_21/1, A_20/1, A_19/1, A_18/1, A_17/1, A_16/1, A_15/1, A_14/1, A_13/1, A_12/1, A_11/1, A_10/1, A_9/1, A_8/1, A_7/1, A_6/1, A_5/1, A_4/1, A_3/1, A_2/1, A_1/1, A_0/1
  A_39/1 -> ALU_SUM_39/2(A_INPUT (1 BIT))
  B_58/1 -> ALU_SUM_58/3(B_INPUT (1 BIT))
  B_20/1 -> ALU_SUM_20/3(B_INPUT (1 BIT))
  ALU_SUM_33/1(ALU_OUT (1 BIT)) -> ALU_OUT_32_BIT1/2(ALU_OUT_1 (1 BIT))
  ALU_SUM_41/1(ALU_OUT (1 BIT)) -> ALU_OUT_32_BIT1/10(ALU_OUT_9 (1 BIT))
  A_58/1 -> ALU_SUM_58/2(A_INPUT (1 BIT))
  ALU_SUM_47/1(ALU_OUT (1 BIT)) -> ALU_OUT_32_BIT1/16(ALU_OUT_15 (1 BIT))
  ALU_SUM_37/2(CARRY_OUT (1 BIT)) -> ALU_SUM_38/1(CARRY_IN (1 BIT))
  B (64 BIT)/1 -> B_58/1, B_60/1, B_62/1, B_63/1, B_61/1, B_59/1, B_57/1, B_56/1, B_55/1, B_54/1, B_53/1, B_52/1, B_51/1, B_50/1, B_49/1, B_48/1, B_47/1, B_46/1, B_45/1, B_44/1, B_43/1, B_42/1, B_41/1, B_40/1, B_39/1, B_38/1, B_37/1, B_36/1, B_35/1, B_34/1, B_33/1, B_32/1, B_31/1, B_30/1, B_29/1, B_28/1, B_27/1, B_26/1, B_25/1, B_24/1, B_23/1, B_22/1, B_21/1, B_20/1, B_19/1, B_18/1, B_17/1, B_16/1, B_15/1, B_14/1, B_13/1, B_12/1, B_11/1, B_10/1, B_9/1, B_8/1, B_7/1, B_6/1, B_5/1, B_4/1, B_3/1, B_2/1, B_1/1, B_0/1
  B_44/1 -> ALU_SUM_44/3(B_INPUT (1 BIT))
  ALU_SUM_59/1(ALU_OUT (1 BIT)) -> ALU_OUT_32_BIT1/28(ALU_OUT_27 (1 BIT))
  ALU_SUM_63/1(ALU_OUT (1 BIT)) -> ALU_OUT_32_BIT1/32(ALU_OUT_31 (1 BIT))
  ALU_SUM_54/2(CARRY_OUT (1 BIT)) -> ALU_SUM_55/1(CARRY_IN (1 BIT))
  ALU_SUM_60/1(ALU_OUT (1 BIT)) -> ALU_OUT_32_BIT1/29(ALU_OUT_28 (1 BIT))
  A_16/1 -> ALU_SUM_16/2(A_INPUT (1 BIT))
  ALU_SUM_24/1(ALU_OUT (1 BIT)) -> ALU_OUT_32_BIT/25(ALU_OUT_24 (1 BIT))
  ALU_SUM_1/1(ALU_OUT (1 BIT)) -> ALU_OUT_32_BIT/2(ALU_OUT_1 (1 BIT))
  ALU_SUM_24/2(CARRY_OUT (1 BIT)) -> ALU_SUM_25/1(CARRY_IN (1 BIT))
  ALU_SUM_16/1(ALU_OUT (1 BIT)) -> ALU_OUT_32_BIT/17(ALU_OUT_16 (1 BIT))
  ALU_SUM_55/2(CARRY_OUT (1 BIT)) -> ALU_SUM_56/1(CARRY_IN (1 BIT))
  ALU_SUM_33/2(CARRY_OUT (1 BIT)) -> ALU_SUM_34/1(CARRY_IN (1 BIT))
  CARRY_IN/1 -> Gateway In12/1
  ALU_SUM_47/2(CARRY_OUT (1 BIT)) -> ALU_SUM_48/1(CARRY_IN (1 BIT))
  A_32/1 -> ALU_SUM_32/2(A_INPUT (1 BIT))
  ALU_SUM_43/1(ALU_OUT (1 BIT)) -> ALU_OUT_32_BIT1/12(ALU_OUT_11 (1 BIT))
  ALU_SUM_34/1(ALU_OUT (1 BIT)) -> ALU_OUT_32_BIT1/3(ALU_OUT_2 (1 BIT))
  A_18/1 -> ALU_SUM_18/2(A_INPUT (1 BIT))
  ALU_SUM_62/2(CARRY_OUT (1 BIT)) -> ALU_SUM_63/1(CARRY_IN (1 BIT))
  ALU_SUM_35/2(CARRY_OUT (1 BIT)) -> ALU_SUM_36/1(CARRY_IN (1 BIT))
  B_0/1 -> ALU_SUM_0/3(B_INPUT (1 BIT))
  ALU_SUM_42/2(CARRY_OUT (1 BIT)) -> ALU_SUM_43/1(CARRY_IN (1 BIT))
  A_3/1 -> ALU_SUM_3/2(A_INPUT (1 BIT))
  B_1/1 -> ALU_SUM_1/3(B_INPUT (1 BIT))
  B_59/1 -> ALU_SUM_59/3(B_INPUT (1 BIT))
  ALU_SUM_28/2(CARRY_OUT (1 BIT)) -> ALU_SUM_29/1(CARRY_IN (1 BIT))
  ALU_SUM_56/1(ALU_OUT (1 BIT)) -> ALU_OUT_32_BIT1/25(ALU_OUT_24 (1 BIT))
  ALU_SUM_25/2(CARRY_OUT (1 BIT)) -> ALU_SUM_26/1(CARRY_IN (1 BIT))
  ALU_SUM_9/1(ALU_OUT (1 BIT)) -> ALU_OUT_32_BIT/10(ALU_OUT_9 (1 BIT))
  A_60/1 -> ALU_SUM_60/2(A_INPUT (1 BIT))
  ALU_SUM_40/1(ALU_OUT (1 BIT)) -> ALU_OUT_32_BIT1/9(ALU_OUT_8 (1 BIT))
  A_56/1 -> ALU_SUM_56/2(A_INPUT (1 BIT))
  ALU_SUM_4/2(CARRY_OUT (1 BIT)) -> ALU_SUM_5/1(CARRY_IN (1 BIT))
  ALU_SUM_10/2(CARRY_OUT (1 BIT)) -> ALU_SUM_11/1(CARRY_IN (1 BIT))
  ALU_SUM_57/1(ALU_OUT (1 BIT)) -> ALU_OUT_32_BIT1/26(ALU_OUT_25 (1 BIT))
  ALU_SUM_22/1(ALU_OUT (1 BIT)) -> ALU_OUT_32_BIT/23(ALU_OUT_22 (1 BIT))
  B_63/1 -> ALU_SUM_63/3(B_INPUT (1 BIT))
  B_27/1 -> ALU_SUM_27/3(B_INPUT (1 BIT))
  A_63/1 -> ALU_SUM_63/2(A_INPUT (1 BIT))
  ALU_SUM_37/1(ALU_OUT (1 BIT)) -> ALU_OUT_32_BIT1/6(ALU_OUT_5 (1 BIT))
  ALU_SUM_45/1(ALU_OUT (1 BIT)) -> ALU_OUT_32_BIT1/14(ALU_OUT_13 (1 BIT))
  ALU_SUM_52/1(ALU_OUT (1 BIT)) -> ALU_OUT_32_BIT1/21(ALU_OUT_20 (1 BIT))
  A_59/1 -> ALU_SUM_59/2(A_INPUT (1 BIT))
  ALU_SUM_53/1(ALU_OUT (1 BIT)) -> ALU_OUT_32_BIT1/22(ALU_OUT_21 (1 BIT))
  B_55/1 -> ALU_SUM_55/3(B_INPUT (1 BIT))
  A_27/1 -> ALU_SUM_27/2(A_INPUT (1 BIT))
  B_62/1 -> ALU_SUM_62/3(B_INPUT (1 BIT))
  A_30/1 -> ALU_SUM_30/2(A_INPUT (1 BIT))
  ALU_SUM_2/1(ALU_OUT (1 BIT)) -> ALU_OUT_32_BIT/3(ALU_OUT_2 (1 BIT))
  B_2/1 -> ALU_SUM_2/3(B_INPUT (1 BIT))
  A_62/1 -> ALU_SUM_62/2(A_INPUT (1 BIT))
  B_28/1 -> ALU_SUM_28/3(B_INPUT (1 BIT))
  ALU_SUM_16/2(CARRY_OUT (1 BIT)) -> ALU_SUM_17/1(CARRY_IN (1 BIT))
  ALU_SUM_53/2(CARRY_OUT (1 BIT)) -> ALU_SUM_54/1(CARRY_IN (1 BIT))
  B_29/1 -> ALU_SUM_29/3(B_INPUT (1 BIT))
  B_30/1 -> ALU_SUM_30/3(B_INPUT (1 BIT))
  A_47/1 -> ALU_SUM_47/2(A_INPUT (1 BIT))
  _Overflow1/1 -> Display1/1
  ALU_SUM_58/2(CARRY_OUT (1 BIT)) -> ALU_SUM_59/1(CARRY_IN (1 BIT))
  ALU_SUM_12/1(ALU_OUT (1 BIT)) -> ALU_OUT_32_BIT/13(ALU_OUT_12 (1 BIT))
  A_19/1 -> ALU_SUM_19/2(A_INPUT (1 BIT))
  ALU_SUM_18/2(CARRY_OUT (1 BIT)) -> ALU_SUM_19/1(CARRY_IN (1 BIT))
  ALU_SUM_44/1(ALU_OUT (1 BIT)) -> ALU_OUT_32_BIT1/13(ALU_OUT_12 (1 BIT))
  ALU_SUM_14/2(CARRY_OUT (1 BIT)) -> ALU_SUM_15/1(CARRY_IN (1 BIT))
  A_54/1 -> ALU_SUM_54/2(A_INPUT (1 BIT))
  ALU_SUM_58/1(ALU_OUT (1 BIT)) -> ALU_OUT_32_BIT1/27(ALU_OUT_26 (1 BIT))
  ALU_SUM_46/1(ALU_OUT (1 BIT)) -> ALU_OUT_32_BIT1/15(ALU_OUT_14 (1 BIT))
  ALU_SUM_28/1(ALU_OUT (1 BIT)) -> ALU_OUT_32_BIT/29(ALU_OUT_28 (1 BIT))
  B_54/1 -> ALU_SUM_54/3(B_INPUT (1 BIT))
  A_55/1 -> ALU_SUM_55/2(A_INPUT (1 BIT))
  A_22/1 -> ALU_SUM_22/2(A_INPUT (1 BIT))
  B_56/1 -> ALU_SUM_56/3(B_INPUT (1 BIT))
  A_5/1 -> ALU_SUM_5/2(A_INPUT (1 BIT))
  A_35/1 -> ALU_SUM_35/2(A_INPUT (1 BIT))
  B_17/1 -> ALU_SUM_17/3(B_INPUT (1 BIT))
  ALU_SUM_12/2(CARRY_OUT (1 BIT)) -> ALU_SUM_13/1(CARRY_IN (1 BIT))
  ALU_SUM_35/1(ALU_OUT (1 BIT)) -> ALU_OUT_32_BIT1/4(ALU_OUT_3 (1 BIT))
  ALU_SUM_11/2(CARRY_OUT (1 BIT)) -> ALU_SUM_12/1(CARRY_IN (1 BIT))
  ALU_SUM_39/2(CARRY_OUT (1 BIT)) -> ALU_SUM_40/1(CARRY_IN (1 BIT))
  ALU_SUM_38/1(ALU_OUT (1 BIT)) -> ALU_OUT_32_BIT1/7(ALU_OUT_6 (1 BIT))
  ALU_OUT_32_BIT1/1(ALU_SUM (32 BIT)) -> Concat1/1
  ALU_SUM_55/1(ALU_OUT (1 BIT)) -> ALU_OUT_32_BIT1/24(ALU_OUT_23 (1 BIT))
  A_36/1 -> ALU_SUM_36/2(A_INPUT (1 BIT))
  ALU_OUT_32_BIT/1(ALU_SUM (32 BIT)) -> Concat1/2
  A_41/1 -> ALU_SUM_41/2(A_INPUT (1 BIT))
  B_50/1 -> ALU_SUM_50/3(B_INPUT (1 BIT))
  A_61/1 -> ALU_SUM_61/2(A_INPUT (1 BIT))
  A_46/1 -> ALU_SUM_46/2(A_INPUT (1 BIT))
  B_25/1 -> ALU_SUM_25/3(B_INPUT (1 BIT))
  B_61/1 -> ALU_SUM_61/3(B_INPUT (1 BIT))
  B_8/1 -> ALU_SUM_8/3(B_INPUT (1 BIT))
  B_45/1 -> ALU_SUM_45/3(B_INPUT (1 BIT))
  B_60/1 -> ALU_SUM_60/3(B_INPUT (1 BIT))
  ALU_SUM_60/2(CARRY_OUT (1 BIT)) -> ALU_SUM_61/1(CARRY_IN (1 BIT))
  B_34/1 -> ALU_SUM_34/3(B_INPUT (1 BIT))
  Concat1/1 -> A+B (64 BIT)/1, _Overflow1/1
  ALU_SUM_14/1(ALU_OUT (1 BIT)) -> ALU_OUT_32_BIT/15(ALU_OUT_14 (1 BIT))
  ALU_SUM_27/2(CARRY_OUT (1 BIT)) -> ALU_SUM_28/1(CARRY_IN (1 BIT))
  ALU_SUM_63/2(CARRY_OUT (1 BIT)) -> _Overflow/1
  B_51/1 -> ALU_SUM_51/3(B_INPUT (1 BIT))
  A_50/1 -> ALU_SUM_50/2(A_INPUT (1 BIT))
  A_51/1 -> ALU_SUM_51/2(A_INPUT (1 BIT))
  ALU_SUM_50/2(CARRY_OUT (1 BIT)) -> ALU_SUM_51/1(CARRY_IN (1 BIT))
  B_5/1 -> ALU_SUM_5/3(B_INPUT (1 BIT))
  B_41/1 -> ALU_SUM_41/3(B_INPUT (1 BIT))
  ALU_SUM_39/1(ALU_OUT (1 BIT)) -> ALU_OUT_32_BIT1/8(ALU_OUT_7 (1 BIT))
  ALU_SUM_19/1(ALU_OUT (1 BIT)) -> ALU_OUT_32_BIT/20(ALU_OUT_19 (1 BIT))
  A_40/1 -> ALU_SUM_40/2(A_INPUT (1 BIT))
  B_35/1 -> ALU_SUM_35/3(B_INPUT (1 BIT))
  B_57/1 -> ALU_SUM_57/3(B_INPUT (1 BIT))
  ALU_SUM_51/2(CARRY_OUT (1 BIT)) -> ALU_SUM_52/1(CARRY_IN (1 BIT))
  ALU_SUM_34/2(CARRY_OUT (1 BIT)) -> ALU_SUM_35/1(CARRY_IN (1 BIT))
  ALU_SUM_18/1(ALU_OUT (1 BIT)) -> ALU_OUT_32_BIT/19(ALU_OUT_18 (1 BIT))
  ALU_SUM_57/2(CARRY_OUT (1 BIT)) -> ALU_SUM_58/1(CARRY_IN (1 BIT))
  ALU_SUM_61/1(ALU_OUT (1 BIT)) -> ALU_OUT_32_BIT1/30(ALU_OUT_29 (1 BIT))
  ALU_SUM_49/1(ALU_OUT (1 BIT)) -> ALU_OUT_32_BIT1/18(ALU_OUT_17 (1 BIT))
  A_8/1 -> ALU_SUM_8/2(A_INPUT (1 BIT))
  ALU_SUM_51/1(ALU_OUT (1 BIT)) -> ALU_OUT_32_BIT1/20(ALU_OUT_19 (1 BIT))
  B_31/1 -> ALU_SUM_31/3(B_INPUT (1 BIT))
  ALU_SUM_15/2(CARRY_OUT (1 BIT)) -> ALU_SUM_16/1(CARRY_IN (1 BIT))
  ALU_SUM_21/1(ALU_OUT (1 BIT)) -> ALU_OUT_32_BIT/22(ALU_OUT_21 (1 BIT))
  ALU_SUM_31/1(ALU_OUT (1 BIT)) -> ALU_OUT_32_BIT/32(ALU_OUT_31 (1 BIT))
  ALU_SUM_32/1(ALU_OUT (1 BIT)) -> ALU_OUT_32_BIT1/1(ALU_OUT_0 (1 BIT))
  B_48/1 -> ALU_SUM_48/3(B_INPUT (1 BIT))
  ALU_SUM_50/1(ALU_OUT (1 BIT)) -> ALU_OUT_32_BIT1/19(ALU_OUT_18 (1 BIT))
  ALU_SUM_48/1(ALU_OUT (1 BIT)) -> ALU_OUT_32_BIT1/17(ALU_OUT_16 (1 BIT))
  A_21/1 -> ALU_SUM_21/2(A_INPUT (1 BIT))
  ALU_SUM_6/2(CARRY_OUT (1 BIT)) -> ALU_SUM_7/1(CARRY_IN (1 BIT))
  ALU_SUM_5/2(CARRY_OUT (1 BIT)) -> ALU_SUM_6/1(CARRY_IN (1 BIT))
  A_53/1 -> ALU_SUM_53/2(A_INPUT (1 BIT))
  ALU_SUM_52/2(CARRY_OUT (1 BIT)) -> ALU_SUM_53/1(CARRY_IN (1 BIT))
  B_52/1 -> ALU_SUM_52/3(B_INPUT (1 BIT))
  B_53/1 -> ALU_SUM_53/3(B_INPUT (1 BIT))
  A_48/1 -> ALU_SUM_48/2(A_INPUT (1 BIT))
  A_52/1 -> ALU_SUM_52/2(A_INPUT (1 BIT))
  B_49/1 -> ALU_SUM_49/3(B_INPUT (1 BIT))
  ALU_SUM_31/2(CARRY_OUT (1 BIT)) -> ALU_SUM_32/1(CARRY_IN (1 BIT))
  B_16/1 -> ALU_SUM_16/3(B_INPUT (1 BIT))
  B_26/1 -> ALU_SUM_26/3(B_INPUT (1 BIT))
  B_42/1 -> ALU_SUM_42/3(B_INPUT (1 BIT))
  ALU_SUM_17/1(ALU_OUT (1 BIT)) -> ALU_OUT_32_BIT/18(ALU_OUT_17 (1 BIT))
  B_47/1 -> ALU_SUM_47/3(B_INPUT (1 BIT))
  A_13/1 -> ALU_SUM_13/2(A_INPUT (1 BIT))
  ALU_SUM_56/2(CARRY_OUT (1 BIT)) -> ALU_SUM_57/1(CARRY_IN (1 BIT))
  ALU_SUM_19/2(CARRY_OUT (1 BIT)) -> ALU_SUM_20/1(CARRY_IN (1 BIT))
  ALU_SUM_3/2(CARRY_OUT (1 BIT)) -> ALU_SUM_4/1(CARRY_IN (1 BIT))
  ALU_SUM_6/1(ALU_OUT (1 BIT)) -> ALU_OUT_32_BIT/7(ALU_OUT_6 (1 BIT))
  ALU_SUM_23/2(CARRY_OUT (1 BIT)) -> ALU_SUM_24/1(CARRY_IN (1 BIT))
  ALU_SUM_46/2(CARRY_OUT (1 BIT)) -> ALU_SUM_47/1(CARRY_IN (1 BIT))
  ALU_SUM_26/2(CARRY_OUT (1 BIT)) -> ALU_SUM_27/1(CARRY_IN (1 BIT))
  A_0/1 -> ALU_SUM_0/2(A_INPUT (1 BIT))
  B_10/1 -> ALU_SUM_10/3(B_INPUT (1 BIT))
  ALU_SUM_41/2(CARRY_OUT (1 BIT)) -> ALU_SUM_42/1(CARRY_IN (1 BIT))
  A_4/1 -> ALU_SUM_4/2(A_INPUT (1 BIT))
  ALU_SUM_44/2(CARRY_OUT (1 BIT)) -> ALU_SUM_45/1(CARRY_IN (1 BIT))
  B_46/1 -> ALU_SUM_46/3(B_INPUT (1 BIT))
  B_3/1 -> ALU_SUM_3/3(B_INPUT (1 BIT))
  ALU_SUM_30/2(CARRY_OUT (1 BIT)) -> ALU_SUM_31/1(CARRY_IN (1 BIT))
  ALU_SUM_29/2(CARRY_OUT (1 BIT)) -> ALU_SUM_30/1(CARRY_IN (1 BIT))
  B_40/1 -> ALU_SUM_40/3(B_INPUT (1 BIT))
  ALU_SUM_26/1(ALU_OUT (1 BIT)) -> ALU_OUT_32_BIT/27(ALU_OUT_26 (1 BIT))
  A_28/1 -> ALU_SUM_28/2(A_INPUT (1 BIT))
  ALU_SUM_20/1(ALU_OUT (1 BIT)) -> ALU_OUT_32_BIT/21(ALU_OUT_20 (1 BIT))
  B_14/1 -> ALU_SUM_14/3(B_INPUT (1 BIT))
  A_1/1 -> ALU_SUM_1/2(A_INPUT (1 BIT))
  A_9/1 -> ALU_SUM_9/2(A_INPUT (1 BIT))
  A_42/1 -> ALU_SUM_42/2(A_INPUT (1 BIT))
  A_43/1 -> ALU_SUM_43/2(A_INPUT (1 BIT))
  ALU_SUM_7/2(CARRY_OUT (1 BIT)) -> ALU_SUM_8/1(CARRY_IN (1 BIT))
  B_19/1 -> ALU_SUM_19/3(B_INPUT (1 BIT))
  A_26/1 -> ALU_SUM_26/2(A_INPUT (1 BIT))
  A_2/1 -> ALU_SUM_2/2(A_INPUT (1 BIT))
  A_24/1 -> ALU_SUM_24/2(A_INPUT (1 BIT))
  A_15/1 -> ALU_SUM_15/2(A_INPUT (1 BIT))
  ALU_SUM_0/2(CARRY_OUT (1 BIT)) -> ALU_SUM_1/1(CARRY_IN (1 BIT))
  B_38/1 -> ALU_SUM_38/3(B_INPUT (1 BIT))
  ALU_SUM_9/2(CARRY_OUT (1 BIT)) -> ALU_SUM_10/1(CARRY_IN (1 BIT))
  ALU_SUM_8/2(CARRY_OUT (1 BIT)) -> ALU_SUM_9/1(CARRY_IN (1 BIT))
  ALU_SUM_1/2(CARRY_OUT (1 BIT)) -> ALU_SUM_2/1(CARRY_IN (1 BIT))
  A_45/1 -> ALU_SUM_45/2(A_INPUT (1 BIT))
  ALU_SUM_2/2(CARRY_OUT (1 BIT)) -> ALU_SUM_3/1(CARRY_IN (1 BIT))
  A_14/1 -> ALU_SUM_14/2(A_INPUT (1 BIT))
  B_22/1 -> ALU_SUM_22/3(B_INPUT (1 BIT))
  B_39/1 -> ALU_SUM_39/3(B_INPUT (1 BIT))
  A_10/1 -> ALU_SUM_10/2(A_INPUT (1 BIT))
  A_38/1 -> ALU_SUM_38/2(A_INPUT (1 BIT))
  ALU_SUM_13/2(CARRY_OUT (1 BIT)) -> ALU_SUM_14/1(CARRY_IN (1 BIT))
  ALU_SUM_32/2(CARRY_OUT (1 BIT)) -> ALU_SUM_33/1(CARRY_IN (1 BIT))
  ALU_SUM_8/1(ALU_OUT (1 BIT)) -> ALU_OUT_32_BIT/9(ALU_OUT_8 (1 BIT))
  ALU_SUM_20/2(CARRY_OUT (1 BIT)) -> ALU_SUM_21/1(CARRY_IN (1 BIT))
  ALU_SUM_22/2(CARRY_OUT (1 BIT)) -> ALU_SUM_23/1(CARRY_IN (1 BIT))
  ALU_SUM_48/2(CARRY_OUT (1 BIT)) -> ALU_SUM_49/1(CARRY_IN (1 BIT))
  ALU_SUM_21/2(CARRY_OUT (1 BIT)) -> ALU_SUM_22/1(CARRY_IN (1 BIT))
  ALU_SUM_17/2(CARRY_OUT (1 BIT)) -> ALU_SUM_18/1(CARRY_IN (1 BIT))
  B_43/1 -> ALU_SUM_43/3(B_INPUT (1 BIT))
  A_17/1 -> ALU_SUM_17/2(A_INPUT (1 BIT))
  A_49/1 -> ALU_SUM_49/2(A_INPUT (1 BIT))
  B_6/1 -> ALU_SUM_6/3(B_INPUT (1 BIT))
  B_18/1 -> ALU_SUM_18/3(B_INPUT (1 BIT))
  Gateway In12/1 -> ALU_SUM_0/1(CARRY_IN (1 BIT))
  B_24/1 -> ALU_SUM_24/3(B_INPUT (1 BIT))
  A_57/1 -> ALU_SUM_57/2(A_INPUT (1 BIT))
  A_25/1 -> ALU_SUM_25/2(A_INPUT (1 BIT))
  A_44/1 -> ALU_SUM_44/2(A_INPUT (1 BIT))
  ALU_SUM_54/1(ALU_OUT (1 BIT)) -> ALU_OUT_32_BIT1/23(ALU_OUT_22 (1 BIT))
  B_13/1 -> ALU_SUM_13/3(B_INPUT (1 BIT))
  B_11/1 -> ALU_SUM_11/3(B_INPUT (1 BIT))
  ALU_SUM_30/1(ALU_OUT (1 BIT)) -> ALU_OUT_32_BIT/31(ALU_OUT_30 (1 BIT))
  A_34/1 -> ALU_SUM_34/2(A_INPUT (1 BIT))
  B_36/1 -> ALU_SUM_36/3(B_INPUT (1 BIT))
  A_31/1 -> ALU_SUM_31/2(A_INPUT (1 BIT))
  A_7/1 -> ALU_SUM_7/2(A_INPUT (1 BIT))
  A_6/1 -> ALU_SUM_6/2(A_INPUT (1 BIT))
  ALU_SUM_10/1(ALU_OUT (1 BIT)) -> ALU_OUT_32_BIT/11(ALU_OUT_10 (1 BIT))
  A_12/1 -> ALU_SUM_12/2(A_INPUT (1 BIT))
  ALU_SUM_15/1(ALU_OUT (1 BIT)) -> ALU_OUT_32_BIT/16(ALU_OUT_15 (1 BIT))
  B_7/1 -> ALU_SUM_7/3(B_INPUT (1 BIT))
  B_15/1 -> ALU_SUM_15/3(B_INPUT (1 BIT))
  _Overflow/1 -> Display72/1
  A_11/1 -> ALU_SUM_11/2(A_INPUT (1 BIT))
  ALU_SUM_49/2(CARRY_OUT (1 BIT)) -> ALU_SUM_50/1(CARRY_IN (1 BIT))
  ALU_SUM_13/1(ALU_OUT (1 BIT)) -> ALU_OUT_32_BIT/14(ALU_OUT_13 (1 BIT))
  ALU_SUM_27/1(ALU_OUT (1 BIT)) -> ALU_OUT_32_BIT/28(ALU_OUT_27 (1 BIT))
  ALU_SUM_59/2(CARRY_OUT (1 BIT)) -> ALU_SUM_60/1(CARRY_IN (1 BIT))
  ALU_SUM_29/1(ALU_OUT (1 BIT)) -> ALU_OUT_32_BIT/30(ALU_OUT_29 (1 BIT))
  B_21/1 -> ALU_SUM_21/3(B_INPUT (1 BIT))
  B_12/1 -> ALU_SUM_12/3(B_INPUT (1 BIT))
  ALU_SUM_36/2(CARRY_OUT (1 BIT)) -> ALU_SUM_37/1(CARRY_IN (1 BIT))
  ALU_SUM_0/1(ALU_OUT (1 BIT)) -> ALU_OUT_32_BIT/1(ALU_OUT_0 (1 BIT))
  ALU_SUM_40/2(CARRY_OUT (1 BIT)) -> ALU_SUM_41/1(CARRY_IN (1 BIT))
  B_33/1 -> ALU_SUM_33/3(B_INPUT (1 BIT))
  B_32/1 -> ALU_SUM_32/3(B_INPUT (1 BIT))
  ALU_SUM_45/2(CARRY_OUT (1 BIT)) -> ALU_SUM_46/1(CARRY_IN (1 BIT))
  A_33/1 -> ALU_SUM_33/2(A_INPUT (1 BIT))
  A_29/1 -> ALU_SUM_29/2(A_INPUT (1 BIT))
  ALU_SUM_3/1(ALU_OUT (1 BIT)) -> ALU_OUT_32_BIT/4(ALU_OUT_3 (1 BIT))
  B_9/1 -> ALU_SUM_9/3(B_INPUT (1 BIT))
  A_20/1 -> ALU_SUM_20/2(A_INPUT (1 BIT))
  A_23/1 -> ALU_SUM_23/2(A_INPUT (1 BIT))
  ALU_SUM_23/1(ALU_OUT (1 BIT)) -> ALU_OUT_32_BIT/24(ALU_OUT_23 (1 BIT))
  B_4/1 -> ALU_SUM_4/3(B_INPUT (1 BIT))
  B_23/1 -> ALU_SUM_23/3(B_INPUT (1 BIT))
  ALU_SUM_4/1(ALU_OUT (1 BIT)) -> ALU_OUT_32_BIT/5(ALU_OUT_4 (1 BIT))
  ALU_SUM_5/1(ALU_OUT (1 BIT)) -> ALU_OUT_32_BIT/6(ALU_OUT_5 (1 BIT))
  ALU_SUM_25/1(ALU_OUT (1 BIT)) -> ALU_OUT_32_BIT/26(ALU_OUT_25 (1 BIT))
  ALU_SUM_11/1(ALU_OUT (1 BIT)) -> ALU_OUT_32_BIT/12(ALU_OUT_11 (1 BIT))
  ALU_SUM_7/1(ALU_OUT (1 BIT)) -> ALU_OUT_32_BIT/8(ALU_OUT_7 (1 BIT))
  ALU_SUM_38/2(CARRY_OUT (1 BIT)) -> ALU_SUM_39/1(CARRY_IN (1 BIT))
  ALU_SUM_42/1(ALU_OUT (1 BIT)) -> ALU_OUT_32_BIT1/11(ALU_OUT_10 (1 BIT))
  B_37/1 -> ALU_SUM_37/3(B_INPUT (1 BIT))
  A_37/1 -> ALU_SUM_37/2(A_INPUT (1 BIT))
  ALU_SUM_43/2(CARRY_OUT (1 BIT)) -> ALU_SUM_44/1(CARRY_IN (1 BIT))
  ALU_SUM_36/1(ALU_OUT (1 BIT)) -> ALU_OUT_32_BIT1/5(ALU_OUT_4 (1 BIT))
